simulink model "matlab_function_heston"  (R2021a)
settings: Solver=FixedStepDiscrete  StartTime=0.0  StopTime=1  FixedStep=dt  RelTol=1e-3
values from neighbouring files (symbols this model uses):
  dt = T / N    (= 0.00396825396825)    [parameters_heston.m]
  kappa = 2    [parameters_heston.m]
  mu = 0.05    [parameters_heston.m]
  S0 = 100    [parameters_heston.m]
  sigma = 0.3    [parameters_heston.m]
  theta = 0.04    [parameters_heston.m]
  v0 = 0.04    [parameters_heston.m]
settings Model: Creator=jonas  LastModifiedBy=jonas
settings DataIOCC: ExternalInput=[t,u]

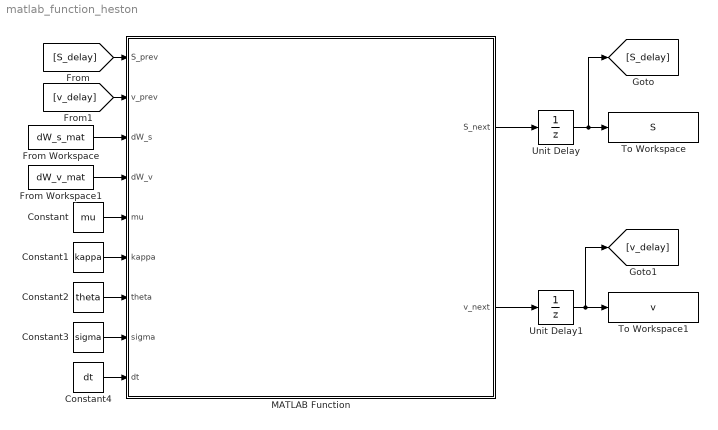
== system matlab_function_heston ==
  Constant : Constant  Value=mu
  Constant1 : Constant  Value=kappa
  Constant2 : Constant  Value=theta
  Constant3 : Constant  Value=sigma
  Constant4 : Constant  Value=dt
  From Workspace : FromWorkspace  VariableName=dW_s_mat
  From Workspace1 : FromWorkspace  VariableName=dW_v_mat
  MATLAB Function : MATLAB Function  TreatAsAtomicUnit=on
  To Workspace : ToWorkspace  VariableName=S  SaveFormat=Structure With Time  SampleTime=-1
  To Workspace1 : ToWorkspace  VariableName=v  SaveFormat=Structure With Time  SampleTime=-1
  Unit Delay : UnitDelay  InitialCondition=S0  SampleTime=dt  HasFrameUpgradeWarning=on
  Unit Delay1 : UnitDelay  InitialCondition=v0  SampleTime=dt  HasFrameUpgradeWarning=on
  wires:
  Constant4/1 -> MATLAB Function/9(dt)
  Constant3/1 -> MATLAB Function/8(sigma)
  Constant2/1 -> MATLAB Function/7(theta)
  Constant1/1 -> MATLAB Function/6(kappa)
  Constant/1 -> MATLAB Function/5(mu)
  From Workspace1/1 -> MATLAB Function/4(dW_v)
  From Workspace/1 -> MATLAB Function/3(dW_s)
  MATLAB Function/1(S_next) -> Unit Delay/1
  MATLAB Function/2(v_next) -> Unit Delay1/1
  [S_delay] -> MATLAB Function/1(S_prev)
  [v_delay] -> MATLAB Function/2(v_prev)
  Unit Delay/1 -> [S_delay], To Workspace/1
  Unit Delay1/1 -> [v_delay], To Workspace1/1

== matlab function matlab_function_heston/MATLAB Function ==
  data: S_prev input; S_next output; v_prev input; dW_s input; dW_v input; mu input; kappa input; theta input; sigma input; dt input; v_next output
function [S_next, v_next] = Heston(S_prev, v_prev, dW_s, dW_v, mu, kappa, theta, sigma, dt)
% Full truncation + log-Euler update (per-step)
% Inputs: scalars (sample-by-sample)
% v_prev could be scalar or vector if multiple sims in one model

% Ensure non-negativity under sqrt
vpos = max(v_prev, 0);

% Variance update (Euler-Maruyama)
dv = kappa.*(theta - vpos).*dt + sigma.*sqrt(vpos).*dW_v;
v_next = v_prev + dv;

% Safety guards
if isnan(v_next) || isinf(v_next)
    v_next = 0;
end
% Boundaries (avoid huge negatives)
if v_next < -1e8
    v_next = 0;
end

% Asset update: log-Euler
drift = (mu - 0.5.*vpos).*dt;
diffusion = sqrt(vpos).*dW_s;
S_next = S_prev .* exp(drift + diffusion);

% Guard S_next
if isnan(S_next) || isinf(S_next) || S_next < 0
    % if weird, fallback to previous
    S_next = max(S_prev, 0);
end
end
